simulink model "Sim46"  (R2019a)
settings: Solver=FixedStepAuto  StartTime=0.0  StopTime=10.0  FixedStep=0.0001  RelTol=1e-3
settings Model: Creator=fbleo  LastModifiedBy=fbleo
settings SolverCC: AlgebraicLoopSolver=LineSearch

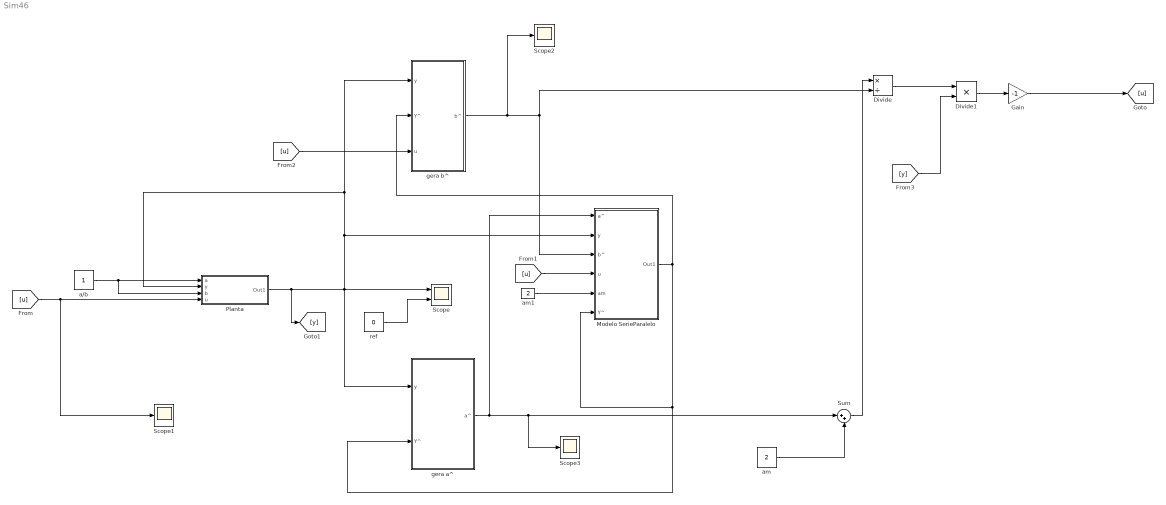
== system Sim46 ==
  Divide : Product  Inputs=*/
  Divide1 : Product  Inputs=**
  Gain : Gain  Gain=-1
  Modelo SerieParalelo : Subsystem
  Planta : Subsystem
  Scope : Scope  NumInputPorts=2
  Scope1 : Scope
  Scope2 : Scope
  Scope3 : Scope
  Sum : Sum  Inputs=|++
  a/b : Constant
  am : Constant  Value=2
  am1 : Constant  Value=2
  gera a^ : Subsystem
  gera b^ : Subsystem
  ref : Constant  Value=0
  wires:
  gera b^/1(b^) -> Scope2/1, Modelo SerieParalelo/3(b^), Divide/2
  [u] -> gera b^/3(u)
  Divide1/1 -> Gain/1
  [y] -> Divide1/2
  [u] -> Scope1/1, Planta/4(u)
  Planta/1(Out1) -> [y], gera a^/1(y), Modelo SerieParalelo/2(y), gera b^/1(y), Planta/2(y), Scope/1
  Gain/1 -> [u]
  gera a^/1(a^) -> Scope3/1, Sum/1, Modelo SerieParalelo/1(a^)
  am/1 -> Sum/2
  [u] -> Modelo SerieParalelo/4(u)
  am1/1 -> Modelo SerieParalelo/5(am)
  Divide/1 -> Divide1/1
  a/b/1 -> Planta/3(b), Planta/1(a)
  Sum/1 -> Divide/1
  Modelo SerieParalelo/1(Out1) -> gera b^/2(Y^), Modelo SerieParalelo/6(Y^), gera a^/2(Y^)
  ref/1 -> Scope/2

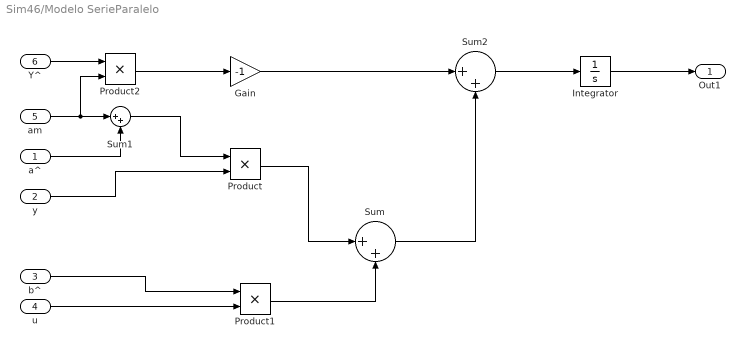
== system Sim46/Modelo SerieParalelo ==
  a^ : Inport
  y : Inport  Port=2
  b^ : Inport  Port=3
  u : Inport  Port=4
  am : Inport  Port=5
  Y^ : Inport  Port=6
  Gain : Gain  Gain=-1
  Integrator : Integrator  InitialCondition=1
  Product : Product
  Product1 : Product
  Product2 : Product
  Sum : Sum  Inputs=|++
  Sum1 : Sum  Inputs=|++
  Sum2 : Sum  Inputs=|++
  Out1 : Outport
  wires:
  a^/1 -> Sum1/2
  y/1 -> Product/2
  Product/1 -> Sum/1
  u/1 -> Product1/2
  b^/1 -> Product1/1
  Product1/1 -> Sum/2
  Sum/1 -> Sum2/2
  Integrator/1 -> Out1/1
  am/1 -> Product2/2, Sum1/1
  Sum1/1 -> Product/1
  Y^/1 -> Product2/1
  Product2/1 -> Gain/1
  Gain/1 -> Sum2/1
  Sum2/1 -> Integrator/1

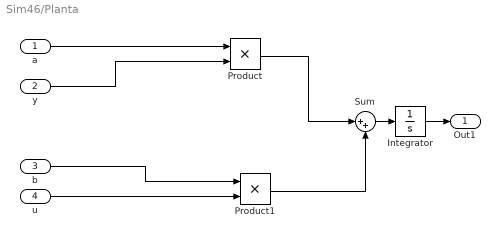
== system Sim46/Planta ==
  a : Inport
  y : Inport  Port=2
  b : Inport  Port=3
  u : Inport  Port=4
  Integrator : Integrator  InitialCondition=0.5
  Product : Product
  Product1 : Product
  Sum : Sum  Inputs=|++
  Out1 : Outport
  wires:
  a/1 -> Product/1
  y/1 -> Product/2
  Product/1 -> Sum/1
  u/1 -> Product1/2
  b/1 -> Product1/1
  Product1/1 -> Sum/2
  Sum/1 -> Integrator/1
  Integrator/1 -> Out1/1

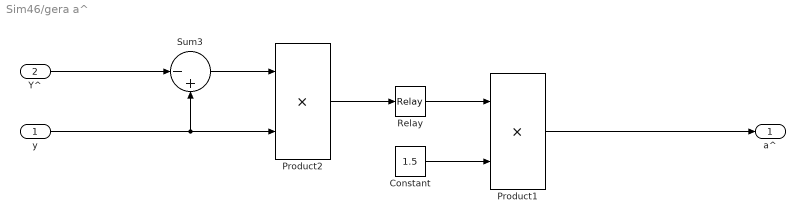
== system Sim46/gera a^ ==
  y : Inport
  Y^ : Inport  Port=2
  Constant : Constant  Value=1.5
  Product1 : Product
  Product2 : Product
  Relay : Relay  OnSwitchValue=0.01  OffSwitchValue=-0.01  OffOutputValue=-1
  Sum3 : Sum  Inputs=|-+
  a^ : Outport
  wires:
  Sum3/1 -> Product2/1
  Y^/1 -> Sum3/1
  y/1 -> Sum3/2, Product2/2
  Product1/1 -> a^/1
  Product2/1 -> Relay/1
  Relay/1 -> Product1/1
  Constant/1 -> Product1/2

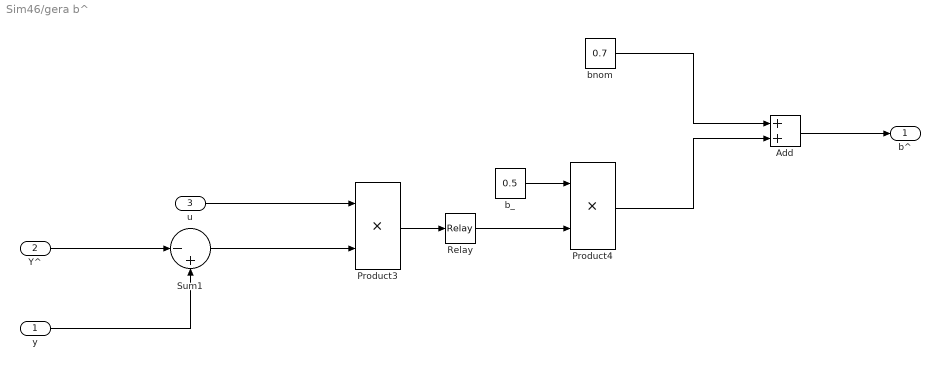
== system Sim46/gera b^ ==
  y : Inport
  Y^ : Inport  Port=2
  u : Inport  Port=3
  Add : Sum
  Product3 : Product
  Product4 : Product
  Relay : Relay  OnSwitchValue=0.01  OffSwitchValue=-0.01  OffOutputValue=-1
  Sum1 : Sum  Inputs=|-+
  b_ : Constant  Value=0.5
  bnom : Constant  Value=0.7
  b^ : Outport
  wires:
  u/1 -> Product3/1
  Y^/1 -> Sum1/1
  y/1 -> Sum1/2
  Sum1/1 -> Product3/2
  Product3/1 -> Relay/1
  b_/1 -> Product4/1
  bnom/1 -> Add/1
  Product4/1 -> Add/2
  Add/1 -> b^/1
  Relay/1 -> Product4/2
